simulink model "HighwayLaneFollowingRRTestBench"  (R2023b)
settings: Solver=ode23tb  StartTime=0  StopTime=1000  FixedStep=Ts  RelTol=1e-3
PostLoadFcn:
  | helperSLHighwayLaneFollowingWithRRSetup()
undefined symbols (not defined in the file or in its folder): assessment, camera, Defined, Ego, Lane, m, n, numTargetActors, Ts, User, v_set, vehicleDetectionRange, vehSim3D
libraries: sim3dautolib x6, roadrunnerscenario x4, simulink x4, trackmetricslib x1, sim3dcameralib x1, sim3dprobsensorlib x1, sim3dlib x1, drivingsim3d x1, dspvision x1, drivingscenarioandsensors x1
CloseFcn:
  | helperSLHighwayLaneFollowingWithRRCleanUp()
settings Model: SILPILSystemUnderTest=refmodels  Creator=The MathWorks, Inc.  LastModifiedBy=varun
settings SolverCC: AlgebraicLoopSolver=TrustRegion  MaxZcPerStep=1
settings DataIOCC: SaveOutput=off  DSMLogging=off  SaveTime=off  ReturnWorkspaceOutputs=off
settings OptimizationCC: ReuseModelBlockBuffer=off
settings DebuggingCC: ParameterPrecisionLossMsg=none  UnconnectedInputMsg=warning  UnconnectedOutputMsg=warning  UnconnectedLineMsg=warning  PregeneratedLibrarySubsystemCodeDiagnostic=none  SubsystemReferenceDiagnosticForUnitTest=warning  ArithmeticOperatorsInVariantConditions=warning
settings HardwareCC: ProdLongLongMode=on
settings ModelReferenceCC: EnableRefExpFcnMdlSchedulingChecks=on
settings SFSimCC: SimUseLocalCustomCode=off
settings RTWCC: RTWUseLocalCustomCode=off  DLArmComputeVersion=19.05
settings GRTTargetCC: RTWCAPISignals=on
settings ConfigComp: CovScope=ReferencedModels  CovIncludeTopModel=off

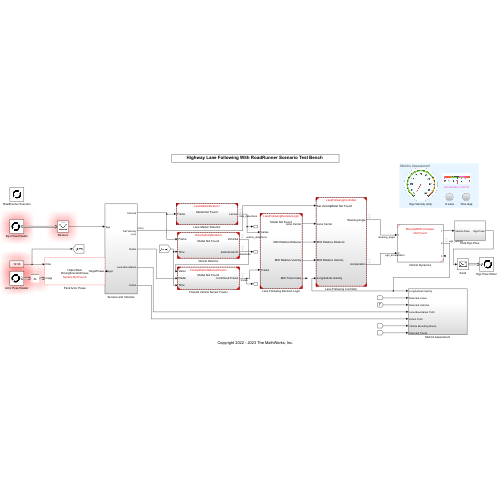
[thumbnail: Simulink's stored preview of the top-level diagram]
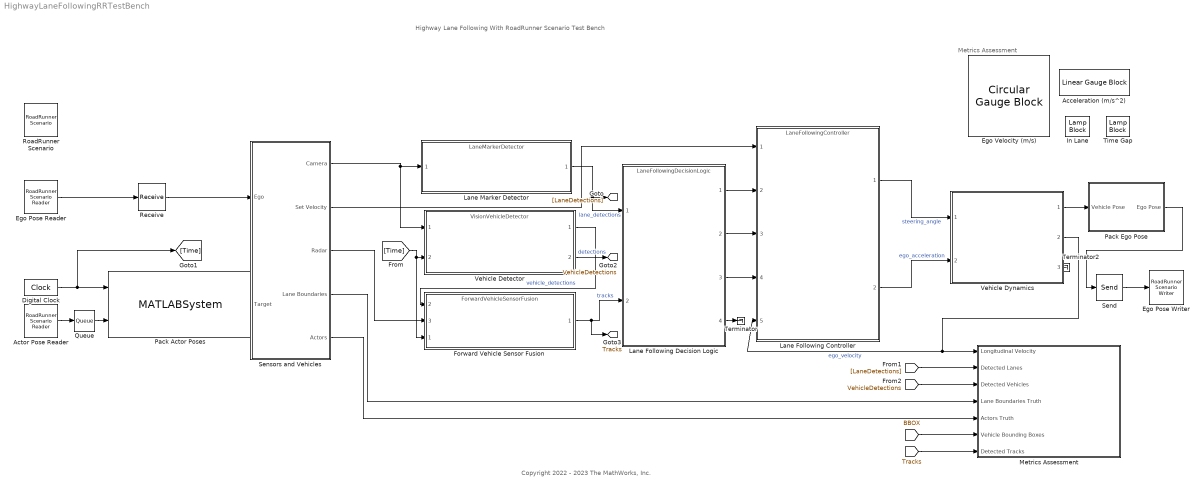
== system HighwayLaneFollowingRRTestBench ==
  note: Highway Lane Following With RoadRunner Scenario Test Bench
  note: Metrics Assessment
  note: Copyright 2022 - 2023 The MathWorks, Inc.
  Acceleration (m/s^2) : LinearGaugeBlock  LabelPosition=Hide  ScaleMin=-6  ScaleMax=6
  Actor Pose Reader : roadrunnerscenario/RoadRunner Scenario Reader  TopicCategory=Actor  ActorCategory=All Types  ActionType=Path Following  EventType=User-Defined  TopicType=Actor Pose (Driving Scenario compatible)  VehicleType=Vehicle Specifications  UserDefinedAction=Action1  UserDefinedEvent=Event1  Filter=None  SensorTopic=Target Poses  LaneBoundaryOutputTopic=Ego-Lane  SensorID=1  SampleTime=Ts
  Digital Clock : DigitalClock  SampleTime=Ts
  Ego Pose Reader : roadrunnerscenario/RoadRunner Scenario Reader  TopicCategory=Actor  ActorCategory=All Types  ActionType=Path Following  EventType=User-Defined  TopicType=Actor Pose (Driving Scenario compatible)  VehicleType=Vehicle Specifications  UserDefinedAction=Action1  UserDefinedEvent=Event1  Filter=Self  SensorTopic=Target Poses  LaneBoundaryOutputTopic=Ego-Lane  SensorID=1  SampleTime=Ts
  Ego Pose Writer : roadrunnerscenario/RoadRunner Scenario Writer  TopicCategory=Actor  ActorCategory=All Types  EventType=Action Complete  UserDefinedEvent=Event1  VehicleType=Vehicle Pose  TopicType=Actor Pose (Driving Scenario compatible)
  Ego Velocity (m/s) : CircularGaugeBlock  LabelPosition=Hide  ScaleMax=50
  Forward Vehicle Sensor Fusion : ModelReference  ModelNameDialog=ForwardVehicleSensorFusion.slx  SimulationMode=Normal  CodeInterface=Top model  ModelReferenceVersion=8.1
      settings: PortSchema="{\"entries\":[{\"content\":{\"sides\":[{\"content\":{\"connectorIds\":[\"In2\",\"In3\",\"In1\"]},\"type\":\"ConnectorPlacement.EquallySpacedRectSide\",\"uuid\":\"7686684e-3ce8-49a8-9c28-78afc562c6cd\"},{\"content\":{\"connectorIds\":[\"Out1\"],\"side\":\"RIGHT\"},\"type\":\"ConnectorPlacement.EquallySpacedRectSide\",\"uuid\":\"c415bca7-2ba8-48d1-9f28-43832dd5ba4e\"},{\"content\":{\"connectorIds\":[],\"side\":\"TOP\"},\"type\":\"ConnectorPlacement.EquallySpacedRectSide\",\"uuid\":\"f22886ed-f0b4-4628-af34-640797a1171b\"}]},\"type\":\"ConnectorPlacement.EquallySpacedConnector\",\"uuid\":\"6b238f4e-3dd4-4f3d-8d3a-ef3e86789fb5\"}],\"packageUris\":[\"http://schema.mathworks.com/mf0/Connector/R2020b\"],\"version\":\"1.0\"}"
  In Lane : LampBlock  LabelPosition=Hide
  Lane Following Controller : ModelReference  ModelNameDialog=LaneFollowingController  SimulationMode=Normal  CodeInterface=Top model  ModelReferenceVersion=8.1
  Lane Following Decision Logic : ModelReference  ModelNameDialog=LaneFollowingDecisionLogic.slx  SimulationMode=Normal  CodeInterface=Top model  ModelReferenceVersion=7.1
  Lane Marker Detector : ModelReference  ModelNameDialog=LaneMarkerDetector.slx  SimulationMode=Normal  CodeInterface=Top model  ModelReferenceVersion=6.1
  Metrics Assessment : Subsystem
  Pack Actor Poses : MATLABSystem  InputPortMessageModes=n,m  System=HelperPackDrivingScenarioPoses  EgoActorID=1  ActorProfiles=actorProfiles  DefaultActorPoses="Simulink.Bus.createMATLABStruct( \"BusActors\" )"
      mask Type: HelperPackDrivingScenarioPoses
      mask Display:
      | disp(['HelperPack' char(10) 'DrivingScenarioPoses']);
      | port_label('input',1,'time');
      | port_label('input',2,'msgs');
      | port_label('output',1,'TargetPoses');
  Pack Ego Pose : Subsystem
  Queue : Queue  InputPortMessageModes=m  OutputPortMessageModes=m  OverwriteOldest=on  Capacity=numTargetActors+2  QueueType=LIFO
  Receive : Receive  InputPortMessageModes=m  UseInternalQueue=off  QueueOverwriting=on  QueueLength=1  QueueType=LIFO  SampleTime=Ts
  RoadRunner Scenario : roadrunnerscenario/RoadRunner Scenario  UserDefinedActions={}  UserDefinedEvents={}
  Send : Send  OutputPortMessageModes=m
  Sensors and Vehicles : Subsystem  VariantControl=1
  Terminator : Terminator
  Terminator2 : Terminator
  Time Gap : LampBlock  LabelPosition=Hide
  Vehicle Detector : ModelReference  ModelNameDialog=VisionVehicleDetector.slx  SimulationMode=Normal  CodeInterface=Top model  ModelReferenceVersion=7.1
  Vehicle Dynamics : Subsystem  VariantControl=Variant2  ReferencedSubsystem=BicycleWithForceInput
  tag scope: Tracks=global, VehicleDetections=global
  wires:
  Ego Pose Reader/1 -> Receive/1
  Lane Following Decision Logic/4 -> Terminator/1
  Digital Clock/1 -> Pack Actor Poses/1, [Time]
  Lane Following Decision Logic/3 -> Lane Following Controller/4
  Vehicle Dynamics/2 -> Lane Following Controller/5, Metrics Assessment/1(Longitudinal Velocity)  "ego_velocity"
  Vehicle Detector/2 -> [VehicleDetections]  "detections"
  Vehicle Detector/1 -> Forward Vehicle Sensor Fusion/2  "vehicle_detections"
  Send/1 -> Ego Pose Writer/1
  Forward Vehicle Sensor Fusion/1 -> [Tracks], Lane Following Decision Logic/2  "tracks"
  Lane Following Decision Logic/2 -> Lane Following Controller/3
  Lane Following Decision Logic/1 -> Lane Following Controller/2
  Lane Following Controller/1 -> Vehicle Dynamics/1  "steering_angle"
  Lane Following Controller/2 -> Vehicle Dynamics/2  "ego_acceleration"
  Sensors and Vehicles/1(Camera) -> Vehicle Detector/1, Lane Marker Detector/1
  Sensors and Vehicles/3(Radar) -> Forward Vehicle Sensor Fusion/3
  Vehicle Dynamics/3 -> Terminator2/1
  Lane Marker Detector/1 -> [LaneDetections], Lane Following Decision Logic/1  "lane_detections"
  Sensors and Vehicles/4(Lane Boundaries) -> Metrics Assessment/4(Lane Boundaries Truth)
  Sensors and Vehicles/2(Set Velocity) -> Lane Following Controller/1
  Vehicle Dynamics/1 -> Pack Ego Pose/1(Vehicle Pose)
  Receive/1 -> Sensors and Vehicles/1(Ego)
  Actor Pose Reader/1 -> Queue/1
  Pack Ego Pose/1(Ego Pose) -> Send/1
  Queue/1 -> Pack Actor Poses/2
  [Time] -> Forward Vehicle Sensor Fusion/1, Vehicle Detector/2
  Pack Actor Poses/1 -> Sensors and Vehicles/2(Target)
  [LaneDetections] -> Metrics Assessment/2(Detected Lanes)
  [VehicleDetections] -> Metrics Assessment/3(Detected Vehicles)
  [Tracks] -> Metrics Assessment/7(Detected Tracks)
  Sensors and Vehicles/5(Actors) -> Metrics Assessment/5(Actors Truth)
  [BBOX] -> Metrics Assessment/6(Vehicle Bounding Boxes)

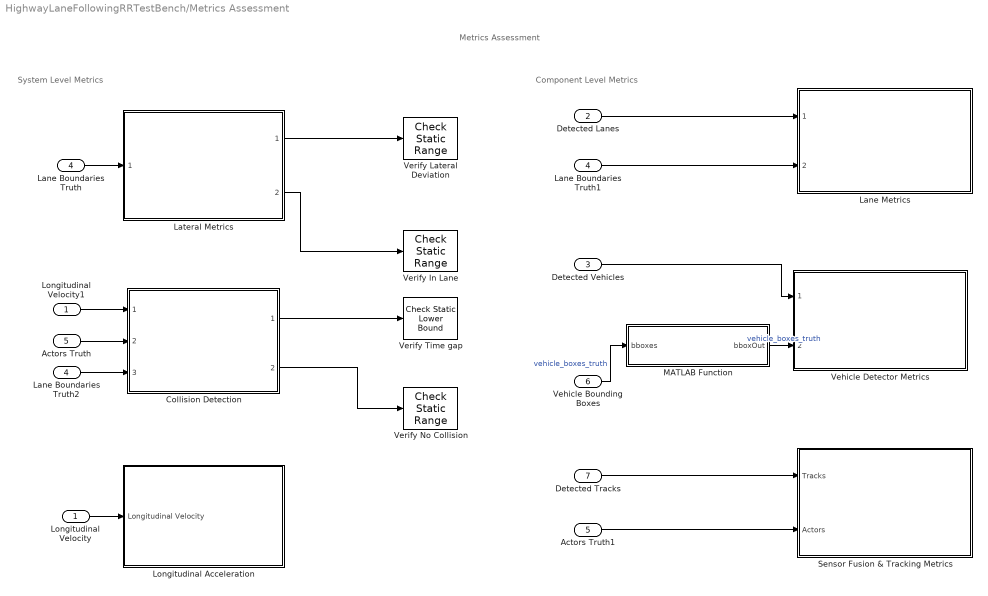
== system HighwayLaneFollowingRRTestBench/Metrics Assessment ==
  note: System Level Metrics
  note: Component Level Metrics
  note: Metrics Assessment
  Longitudinal Velocity : Inport
  Detected Lanes : Inport  Port=2
  Detected Vehicles : Inport  Port=3
  Lane Boundaries Truth : Inport  Port=4
  Actors Truth : Inport  Port=5
  Vehicle Bounding Boxes : Inport  Port=6
  Detected Tracks : Inport  Port=7
  " Vehicle Detector Metrics" : Subsystem  ReferencedSubsystem=VehicleDetectorMetrics
  Actors Truth1 : InportShadow  Port=5
  Collision Detection : Subsystem  ReferencedSubsystem=CollisionDetection
  Lane Boundaries Truth1 : InportShadow  Port=4
  Lane Boundaries Truth2 : InportShadow  Port=4
  Lane Metrics : Subsystem  ReferencedSubsystem=LaneMetrics
  Lateral Metrics : Subsystem  ReferencedSubsystem=LateralMetrics
  Longitudinal Acceleration : Subsystem
  Longitudinal Velocity1 : InportShadow
  MATLAB Function : MATLAB Function  TreatAsAtomicUnit=on  mask{camera=camera, range=vehicleDetectionRange}
  Sensor Fusion & Tracking Metrics : Subsystem
  Verify In Lane : simulink/Model Verification/Check  Static Range  Description=1 <= u <= 1  max=1  max_included=on  min=1  min_included=on  enabled=on  stopWhenAssertionFail=on  export=off  icon=graphic
  Verify Lateral Deviation : simulink/Model Verification/Check  Static Range  Description=-assessment.LateralDeviationMax <= u <= assessment.LateralDeviationMax  max=assessment.LateralDeviationMax  max_included=on  min=-assessment.LateralDeviationMax  min_included=on  enabled=on  stopWhenAssertionFail=on  export=off  icon=graphic
      settings: AttributesFormatString=|
      | ---------------------------------------
      | max = %<max>
      | min = %<min>
  Verify No Collision : simulink/Model Verification/Check  Static Range  Description=0 <= u <= 0  max=0  max_included=on  min=0  min_included=on  enabled=on  stopWhenAssertionFail=on  export=off  icon=graphic
  Verify Time gap : simulink/Model Verification/Check Static  Lower Bound  Description=assessment.TimeGap <= u  min=assessment.TimeGap  min_included=on  enabled=on  stopWhenAssertionFail=on  export=off  icon=graphic
      settings: AttributesFormatString=|
      | ---------------------------------------
      | min = %<min>
  wires:
  Lane Boundaries Truth/1 -> Lateral Metrics/1
  Collision Detection/1 -> Verify Time gap/1
  Lateral Metrics/1 -> Verify Lateral Deviation/1
  Collision Detection/2 -> Verify No Collision/1
  Longitudinal Velocity/1 -> Longitudinal Acceleration/1(Longitudinal Velocity)
  Actors Truth/1 -> Collision Detection/2
  Lateral Metrics/2 -> Verify In Lane/1
  Lane Boundaries Truth2/1 -> Collision Detection/3
  Detected Lanes/1 -> Lane Metrics/1
  Detected Vehicles/1 -> " Vehicle Detector Metrics"/1
  Vehicle Bounding Boxes/1 -> MATLAB Function/1(bboxes)  "vehicle_boxes_truth"
  Lane Boundaries Truth1/1 -> Lane Metrics/2
  Longitudinal Velocity1/1 -> Collision Detection/1
  MATLAB Function/1(bboxOut) -> " Vehicle Detector Metrics"/2  "vehicle_boxes_truth"
  Detected Tracks/1 -> Sensor Fusion & Tracking Metrics/1(Tracks)
  Actors Truth1/1 -> Sensor Fusion & Tracking Metrics/2(Actors)

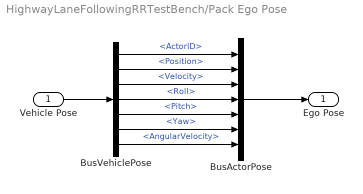
== system HighwayLaneFollowingRRTestBench/Pack Ego Pose ==
  Vehicle Pose : Inport
  BusActorPose : BusCreator  Inputs=7  OutDataTypeStr=Bus: BusActorPose  NonVirtualBus=on
      settings: InheritFromInputs=off
  BusVehiclePose : BusSelector  OutputSignals=ActorID,Position,Velocity,Roll,Pitch,Yaw,AngularVelocity
  Ego Pose : Outport
  wires:
  BusVehiclePose/4 -> BusActorPose/4  "<Roll>"
  BusVehiclePose/3 -> BusActorPose/3  "<Velocity>"
  BusVehiclePose/1 -> BusActorPose/1  "<ActorID>"
  BusVehiclePose/2 -> BusActorPose/2  "<Position>"
  BusVehiclePose/7 -> BusActorPose/7  "<AngularVelocity>"
  BusVehiclePose/6 -> BusActorPose/6  "<Yaw>"
  BusVehiclePose/5 -> BusActorPose/5  "<Pitch>"
  Vehicle Pose/1 -> BusVehiclePose/1
  BusActorPose/1 -> Ego Pose/1

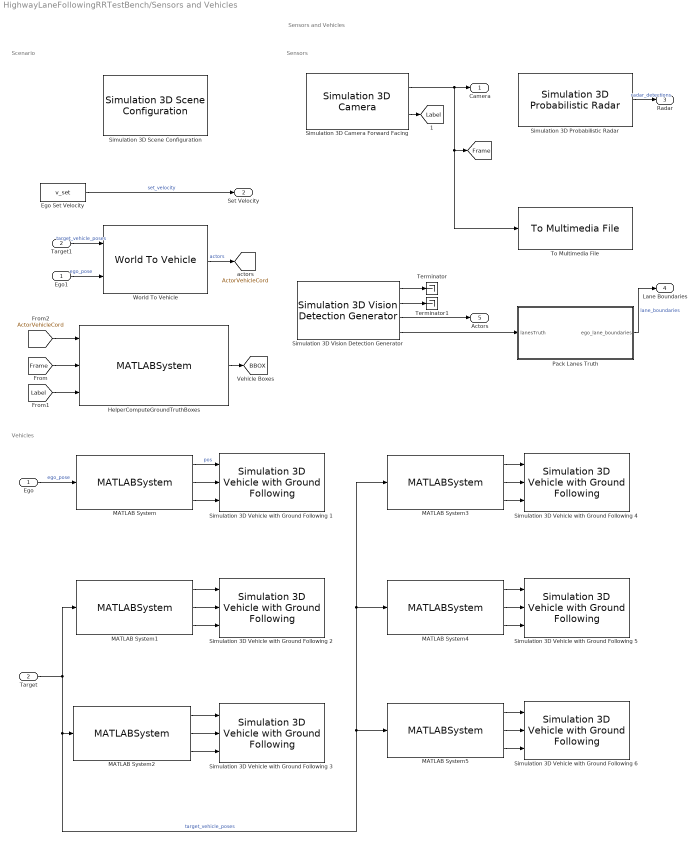
== system HighwayLaneFollowingRRTestBench/Sensors and Vehicles ==
  note: Scenario
  note: Vehicles
  note: Sensors and Vehicles
  note: Sensors
  Ego : Inport
  Target : Inport  Port=2
  Ego Set Velocity : Constant  Value=v_set  SampleTime=Ts
  Ego1 : InportShadow
  HelperComputeGroundTruthBoxes : MATLABSystem  System=HelperComputeGroundTruthBoxes  VehicleDimensions=actorDimensions  Camera=camera  SimulateUsing=Interpreted execution
      mask Type: HelperComputeGroundTruthBoxes
      mask Display:
      | disp('HelperComputeGroundTruthBoxes');
      | port_label('input',1,'actorPositions');
      | port_label('input',2,'frame');
      | port_label('input',3,'labelledFrame');
      | port_label('output',1,'BBoxes');
  MATLAB System : MATLABSystem  System=HelperConvertDSPoseToSim3D  ActorProfiles=actorProfiles  ActorIDToConvert=1  SimulateUsing=Interpreted execution
      mask Type: HelperConvertDSPoseToSim3D
      mask Display:
      | disp(['HelperConvert' char(10) 'DSPoseToSim3D' char(10) 'ActorID: 1']);
      | port_label('input',1,'Actor');
      | port_label('output',1,'X');
      | port_label('output',2,'Y');
      | port_label('output',3,'Yaw');
  MATLAB System1 : MATLABSystem  System=HelperConvertDSPoseToSim3D  ActorProfiles=actorProfiles  ActorIDToConvert=2  SimulateUsing=Interpreted execution
      mask Type: HelperConvertDSPoseToSim3D
      mask Display:
      | disp(['HelperConvert' char(10) 'DSPoseToSim3D' char(10) 'ActorID: 2']);
      | port_label('input',1,'Actor');
      | port_label('output',1,'X');
      | port_label('output',2,'Y');
      | port_label('output',3,'Yaw');
  MATLAB System2 : MATLABSystem  System=HelperConvertDSPoseToSim3D  ActorProfiles=actorProfiles  ActorIDToConvert=3  SimulateUsing=Interpreted execution
      mask Type: HelperConvertDSPoseToSim3D
      mask Display:
      | disp(['HelperConvert' char(10) 'DSPoseToSim3D' char(10) 'ActorID: 3']);
      | port_label('input',1,'Actor');
      | port_label('output',1,'X');
      | port_label('output',2,'Y');
      | port_label('output',3,'Yaw');
  MATLAB System3 : MATLABSystem  System=HelperConvertDSPoseToSim3D  ActorProfiles=actorProfiles  ActorIDToConvert=4  SimulateUsing=Interpreted execution
      mask Type: HelperConvertDSPoseToSim3D
      mask Display:
      | disp(['HelperConvert' char(10) 'DSPoseToSim3D' char(10) 'ActorID: 4']);
      | port_label('input',1,'Actor');
      | port_label('output',1,'X');
      | port_label('output',2,'Y');
      | port_label('output',3,'Yaw');
  MATLAB System4 : MATLABSystem  System=HelperConvertDSPoseToSim3D  ActorProfiles=actorProfiles  ActorIDToConvert=5  SimulateUsing=Interpreted execution
      mask Type: HelperConvertDSPoseToSim3D
      mask Display:
      | disp(['HelperConvert' char(10) 'DSPoseToSim3D' char(10) 'ActorID: 5']);
      | port_label('input',1,'Actor');
      | port_label('output',1,'X');
      | port_label('output',2,'Y');
      | port_label('output',3,'Yaw');
  MATLAB System5 : MATLABSystem  System=HelperConvertDSPoseToSim3D  ActorProfiles=actorProfiles  ActorIDToConvert=6  SimulateUsing=Interpreted execution
      mask Type: HelperConvertDSPoseToSim3D
      mask Display:
      | disp(['HelperConvert' char(10) 'DSPoseToSim3D' char(10) 'ActorID: 6']);
      | port_label('input',1,'Actor');
      | port_label('output',1,'X');
      | port_label('output',2,'Y');
      | port_label('output',3,'Yaw');
  Pack Lanes Truth : MATLAB Function  TreatAsAtomicUnit=on  mask{detStructObj=Simulink.Bus.createMATLABStruct('LaneSensor'), boundariesStructObj=Simulink.Bus.createMATLABStruct('BusLaneBoundaries')}
      mask prompts: detStructObj "Output lane detections struct"; boundariesStructObj "Output lane boundaries struct"
  Simulation 3D Camera Forward Facing : sim3dcameralib/Simulation 3D Camera  Priority=1  sensorTag=Sim3dSensor1  sensorId=1  sensorName=Sim3dSensor1  vehTagList={'Scene Origin';'SimulinkVehicle1';'SimulinkVehicle2';'SimulinkVehicle3';'SimulinkVehicle4';'SimulinkVehicle5';'SimulinkVehicle6'}  vehTag=Scene Origin  mountLoc=Origin  offsetFlag=on  tmountOffset=[0,-1,1]  extTmount=off  rmountOffset=[0,0,-90]  extRmount=off  FocalLength=camera.FocalLength  OpticalCenter=camera.PrincipalPoint  ImageSize=camera.ImageSize  RadialDistortion=[0, 0]  TangentialDistortion=[0, 0]  SensorSkew=0  DepthOutportEnabled=off  SemanticOutportEnabled=on  TransformOutportEnabled=off  SampleTime=-1  mountPoint=[0 1 1]  mountOrientation=[0 0 90]  aMode=3  ID=1
      settings: LibrarySourceBlock=drivingsim3d/Simulation 3D Camera
      settings: AttributesFormatString=|
      | -------------------------------------
      | ImageSize = %<ImageSize>
      | OpticalCenter = %<OpticalCenter>
      | FocalLength = %<FocalLength>
      | RadialDistortion = %<RadialDistortion>
      | mountLoc = %<mountLoc>
      | tmountOffset = %<tmountOffset>
      | rmountOffset = %<rmountOffset>
      | Priority = %<Priority>
  Simulation 3D Probabilistic Radar : sim3dprobsensorlib/Simulation 3D Probabilistic Radar  Priority=1  sensorTag=Sim3dSensor2  sensorId=2  sensorName=Sim3dSensor2  vehTagList={'Scene Origin';'SimulinkVehicle1';'SimulinkVehicle2';'SimulinkVehicle3';'SimulinkVehicle4';'SimulinkVehicle5';'SimulinkVehicle6'}  vehTag=SimulinkVehicle1  mountLoc=Origin  offsetFlag=on  tmountOffset=radar.PositionSim3d  rmountOffset=radar.Rotation  AzimuthResolution=0.8  ElevationResolution=8  RangeResolution=1  RangeRateResolution=1  AzimuthBiasFraction=0.1  ElevationBiasFraction=0.1  RangeBiasFraction=0.05  RangeRateBiasFraction=0.05  FieldOfView=radar.FieldOfView  DetectionRange=radar.DetectionRanges  RangeRateLimits=[ -100, 100 ]  DetectionProbability=0.9  FalseAlarmRate=1e-6  ReferenceRange=150  ReferenceRCS=0  HasElevation=off  HasRangeRate=on  HasNoise=off  HasFalseAlarms=off  InitialSeedSource=Repeatable  InitialSeed=0  MaxNumDetections=50  DetectionCoordinates=Sensor spherical  SpecifyOutputBusName=off  BusName=BusSimulation3DRadarTruthSensor  SampleTime=-1  mountPoint=[0 0 1]  mountOrientation=[0 0 0]  aMode=3  ID=2
      settings: LibrarySourceBlock=drivingsim3d/Simulation 3D Probabilistic Radar
      settings: AttributesFormatString=|
      | -------------------------------------
      | FieldOfView = %<FieldOfView>
      | AzimuthResolution = %<AzimuthResolution>
      | DetectionCoordinates = %<DetectionCoordinates>
      | mountLoc = %<mountLoc>
      | tmountOffset = %<tmountOffset>
      | rmountOffset = %<rmountOffset>
      | Priority = %<Priority>
  Simulation 3D Scene Configuration : sim3dlib/Simulation 3D Scene Configuration  Priority=0  ProjectFormat=RoadRunner  SceneDesc=Large parking lot  ProjectName=C:\Program Files\MATLAB\R2023b\toolbox\shared\sim3d_projects\automotive_project_windows\UE\WindowsNoEditor\VehicleSimulation.exe  ScenePath=/Game/Maps/HwStrght  RoadRunnerProjectPath=C:\Users\varun\ME599\AutoPark\AutoPark\Exports\AutoPark.xosc  EnableOpenDRIVE=off  vehTagList={'Custom';'Scene Origin';'SimulinkVehicle1';'SimulinkVehicle2';'SimulinkVehicle3';'SimulinkVehicle4';'SimulinkVehicle5';'SimulinkVehicle6'}  vehTag=Scene Origin  FreeCameraInitialTranslation=[0, 0, 0]  FreeCameraDefaultInitialTranslation=[-6, 0, 2]  FreeCameraInitialRotation=[0, 0, 0]  FreeCameraDefaultInitialRotation=[0, -15, 0]  OpVisEn=off  Ts=Ts  EnableWindow=on  EnableRemoteAccess=off  EnableWeather=off  SunAltitude=40.0  SunAzimuth=90  clouds=10  wind=1  fog=0  rain=0  EnableGeospatial=off  OriginHeight=200  OriginLatitude=40.744652  OriginLongitude=-73.988864  MapStyle=Aerial  AdditionalAssetIDs=[]  UseAdvancedSunSky=off  SolarTime=11  TimeZone=-5  Day=21  Month=9  Year=2022  UseDaylightSavingTime=on  DSTStartDay=10  DSTStartMonth=3  DSTEndDay=3  DSTEndMonth=11  DSTSwitchHour=2  sensorTag=MainCamera3  sensorId=3  sensorName=MainCamera3  mountLoc=Origin  offsetFlag=off  tmountOffset=[0, 0, 0]  rmountOffset=[0, 0, 0]  HorizontalResolution=1280  VerticalResolution=720  HorizontalFOV=60  mountPoint=[0 0 0]  mountOrientation=[0 0 0]  aMode=3  ID=3  GeoTrigger=Inactive
      settings: LibrarySourceBlock=drivingsim3d/Simulation 3D Scene Configuration
      settings: AttributesFormatString=|
      | -------------------------------------
      | SceneName = %<SceneDesc>
      | Priority = %<Priority>
  Simulation 3D Vehicle with Ground Following 1 : sim3dautolib/Simulation 3D Vehicle with Ground Following  Priority=-1  PassVehMesh=Sedan  MeshPath=/MathWorksSimulation/Vehicles/Muscle/Meshes/SK_MuscleCar.SK_MuscleCar  TrackWidth=1.9  WheelBase=3  WheelRadius=0.35  VehColor=Blue  InitialPos=vehSim3D(1).InitialPos  InitialRot=vehSim3D(1).InitialRot  ActorName=SimulinkVehicle1  SampleTime=-1  ActorType=SimulinkVehicle  ID=1  aMode=3  ActorTag=SimulinkVehicle1  CoordinateScheme=ISO  VehLightsControl=off  HeadlightColor=[ 1, 1, 1 ]  HighBeamIntensity=100000  LowBeamIntensity=60000  HighBeamConeAngle=70  LowBeamConeAngle=70  LeftHeadlightOrientation=[ 0, 0 ]  RightHeadlightOrientation=[ 0, 0 ]  BrakelightIntensity=500  ReverselightIntensity=500  SignallightIntensity=500  SignallightPeriod=1  SignalPulseWidth=50  TransformOutportEnabled=off
      settings: LibrarySourceBlock=drivingsim3d/Simulation 3D Vehicle with Ground Following
      settings: AttributesFormatString=|
      | --------------------------------------
      | ActorName = %<ActorName>
      | PassVehMesh = %<PassVehMesh>
      | VehColor = %<VehColor>
      | InitialPos = %<InitialPos>
      | InitialRot = %<InitialRot>
      | Priority = %<Priority>
  Simulation 3D Vehicle with Ground Following 2 : sim3dautolib/Simulation 3D Vehicle with Ground Following  Priority=-1  PassVehMesh=Sedan  MeshPath=/MathWorksSimulation/Vehicles/Muscle/Meshes/SK_MuscleCar.SK_MuscleCar  TrackWidth=1.9  WheelBase=3  WheelRadius=0.35  VehColor=Red  InitialPos=vehSim3D(2).InitialPos  InitialRot=vehSim3D(2).InitialRot  ActorName=SimulinkVehicle2  SampleTime=-1  ActorType=SimulinkVehicle  ID=2  aMode=3  ActorTag=SimulinkVehicle2  CoordinateScheme=ISO  VehLightsControl=off  HeadlightColor=[ 1, 1, 1 ]  HighBeamIntensity=100000  LowBeamIntensity=60000  HighBeamConeAngle=70  LowBeamConeAngle=70  LeftHeadlightOrientation=[ 0, 0 ]  RightHeadlightOrientation=[ 0, 0 ]  BrakelightIntensity=500  ReverselightIntensity=500  SignallightIntensity=500  SignallightPeriod=1  SignalPulseWidth=50  TransformOutportEnabled=off
      settings: LibrarySourceBlock=drivingsim3d/Simulation 3D Vehicle with Ground Following
      settings: AttributesFormatString=|
      | --------------------------------------
      | ActorName = %<ActorName>
      | PassVehMesh = %<PassVehMesh>
      | VehColor = %<VehColor>
      | InitialPos = %<InitialPos>
      | InitialRot = %<InitialRot>
      | Priority = %<Priority>
  Simulation 3D Vehicle with Ground Following 3 : sim3dautolib/Simulation 3D Vehicle with Ground Following  Priority=-1  PassVehMesh=Sedan  MeshPath=/MathWorksSimulation/Vehicles/Muscle/Meshes/SK_MuscleCar.SK_MuscleCar  TrackWidth=1.9  WheelBase=3  WheelRadius=0.35  VehColor=Black  InitialPos=vehSim3D(3).InitialPos  InitialRot=vehSim3D(3).InitialRot  ActorName=SimulinkVehicle3  SampleTime=-1  ActorType=SimulinkVehicle  ID=3  aMode=3  ActorTag=SimulinkVehicle3  CoordinateScheme=ISO  VehLightsControl=off  HeadlightColor=[ 1, 1, 1 ]  HighBeamIntensity=100000  LowBeamIntensity=60000  HighBeamConeAngle=70  LowBeamConeAngle=70  LeftHeadlightOrientation=[ 0, 0 ]  RightHeadlightOrientation=[ 0, 0 ]  BrakelightIntensity=500  ReverselightIntensity=500  SignallightIntensity=500  SignallightPeriod=1  SignalPulseWidth=50  TransformOutportEnabled=off
      settings: LibrarySourceBlock=drivingsim3d/Simulation 3D Vehicle with Ground Following
      settings: AttributesFormatString=|
      | --------------------------------------
      | ActorName = %<ActorName>
      | PassVehMesh = %<PassVehMesh>
      | VehColor = %<VehColor>
      | InitialPos = %<InitialPos>
      | InitialRot = %<InitialRot>
      | Priority = %<Priority>
  Simulation 3D Vehicle with Ground Following 4 : sim3dautolib/Simulation 3D Vehicle with Ground Following  Priority=-1  PassVehMesh=Sedan  MeshPath=/MathWorksSimulation/Vehicles/Muscle/Meshes/SK_MuscleCar.SK_MuscleCar  TrackWidth=1.9  WheelBase=3  WheelRadius=0.35  VehColor=Orange  InitialPos=vehSim3D(4).InitialPos  InitialRot=vehSim3D(4).InitialRot  ActorName=SimulinkVehicle4  SampleTime=-1  ActorType=SimulinkVehicle  ID=4  aMode=3  ActorTag=SimulinkVehicle4  CoordinateScheme=ISO  VehLightsControl=off  HeadlightColor=[ 1, 1, 1 ]  HighBeamIntensity=100000  LowBeamIntensity=60000  HighBeamConeAngle=70  LowBeamConeAngle=70  LeftHeadlightOrientation=[ 0, 0 ]  RightHeadlightOrientation=[ 0, 0 ]  BrakelightIntensity=500  ReverselightIntensity=500  SignallightIntensity=500  SignallightPeriod=1  SignalPulseWidth=50  TransformOutportEnabled=off
      settings: LibrarySourceBlock=drivingsim3d/Simulation 3D Vehicle with Ground Following
      settings: AttributesFormatString=|
      | --------------------------------------
      | ActorName = %<ActorName>
      | PassVehMesh = %<PassVehMesh>
      | VehColor = %<VehColor>
      | InitialPos = %<InitialPos>
      | InitialRot = %<InitialRot>
      | Priority = %<Priority>
  Simulation 3D Vehicle with Ground Following 5 : sim3dautolib/Simulation 3D Vehicle with Ground Following  Priority=-1  PassVehMesh=Sedan  MeshPath=/MathWorksSimulation/Vehicles/Muscle/Meshes/SK_MuscleCar.SK_MuscleCar  TrackWidth=1.9  WheelBase=3  WheelRadius=0.35  VehColor=Green  InitialPos=vehSim3D(5).InitialPos  InitialRot=vehSim3D(5).InitialRot  ActorName=SimulinkVehicle5  SampleTime=-1  ActorType=SimulinkVehicle  ID=5  aMode=3  ActorTag=SimulinkVehicle5  CoordinateScheme=ISO  VehLightsControl=off  HeadlightColor=[ 1, 1, 1 ]  HighBeamIntensity=100000  LowBeamIntensity=60000  HighBeamConeAngle=70  LowBeamConeAngle=70  LeftHeadlightOrientation=[ 0, 0 ]  RightHeadlightOrientation=[ 0, 0 ]  BrakelightIntensity=500  ReverselightIntensity=500  SignallightIntensity=500  SignallightPeriod=1  SignalPulseWidth=50  TransformOutportEnabled=off
      settings: LibrarySourceBlock=drivingsim3d/Simulation 3D Vehicle with Ground Following
      settings: AttributesFormatString=|
      | --------------------------------------
      | ActorName = %<ActorName>
      | PassVehMesh = %<PassVehMesh>
      | VehColor = %<VehColor>
      | InitialPos = %<InitialPos>
      | InitialRot = %<InitialRot>
      | Priority = %<Priority>
  Simulation 3D Vehicle with Ground Following 6 : sim3dautolib/Simulation 3D Vehicle with Ground Following  Priority=-1  PassVehMesh=Sedan  MeshPath=/MathWorksSimulation/Vehicles/Muscle/Meshes/SK_MuscleCar.SK_MuscleCar  TrackWidth=1.9  WheelBase=3  WheelRadius=0.35  VehColor=Blue  InitialPos=vehSim3D(6).InitialPos  InitialRot=vehSim3D(6).InitialRot  ActorName=SimulinkVehicle6  SampleTime=-1  ActorType=SimulinkVehicle  ID=6  aMode=3  ActorTag=SimulinkVehicle6  CoordinateScheme=ISO  VehLightsControl=off  HeadlightColor=[ 1, 1, 1 ]  HighBeamIntensity=100000  LowBeamIntensity=60000  HighBeamConeAngle=70  LowBeamConeAngle=70  LeftHeadlightOrientation=[ 0, 0 ]  RightHeadlightOrientation=[ 0, 0 ]  BrakelightIntensity=500  ReverselightIntensity=500  SignallightIntensity=500  SignallightPeriod=1  SignalPulseWidth=50  TransformOutportEnabled=off
      settings: LibrarySourceBlock=drivingsim3d/Simulation 3D Vehicle with Ground Following
      settings: AttributesFormatString=|
      | --------------------------------------
      | ActorName = %<ActorName>
      | PassVehMesh = %<PassVehMesh>
      | VehColor = %<VehColor>
      | InitialPos = %<InitialPos>
      | InitialRot = %<InitialRot>
      | Priority = %<Priority>
  Simulation 3D Vision Detection Generator : drivingsim3d/Simulation 3D Vision Detection Generator  Priority=1  VariantControl=Choice  sensorTag=Sim3dSensor255  sensorId=3  sensorName=Sim3dSensor3  vehTagList={'Scene Origin';'SimulinkVehicle1';'SimulinkVehicle2';'SimulinkVehicle3';'SimulinkVehicle4';'SimulinkVehicle5';'SimulinkVehicle6'}  vehTag=SimulinkVehicle1  mountLoc=Origin  offsetFlag=on  tmountOffset=[0,-1,1]  rmountOffset=[0,0,0]  DetectorOutput=Lanes and objects  MaxNumDetections=5  MaxNumLanes=30  laneSampleDistances=0:0.5:70  BusNameSource=Property  BusName=BusObjectDetections  BusName2Source=Property  BusName2=BusLaneDetections  MaxRange=camera.DetectionRanges(2)  BoundingBoxAccuracy=5  ProcessNoiseIntensity=5  MaxSpeed=50  MaxAllowedOcclusion=0.5  MinObjectImageSize=camera.MinObjectImageSize  DetectionProbability=1  FalsePositivesPerImage=0  MinLaneImageSize=[ 20, 3 ]  LaneBoundaryAccuracy=3  HasNoise=off  InitialSeedSource=Repeatable  InitialSeed=1  uniqueActorIdentifier=[]  actorClassInteger=0  cuboidLength=4.7  cuboidWidth=1.8  cuboidHeight=1.4  rotationalCenter={[-1.35, 0, 0]}  focalLength=camera.FocalLength  opticalCenter=camera.PrincipalPoint  imageSize=camera.ImageSize  radialDistortionCoefficients=[0, 0]  tangentialDistortionCoefficients=[0, 0]  cameraAxisSkew=0  actorTruthOutportEnabled=on  laneTruthOutportEnabled=on  SampleTime=-1  checkedSampleTime=0.1  mountPoint=[0 1 1]  mountOrientation=[0 0 0]  aMode=3  ID=3
      settings: AttributesFormatString=|
      | imageSize = %<imageSize>
      | opticalCenter = %<opticalCenter>
      | focalLength = %<focalLength>
      | radialDistortionCoefficients = %<radialDistortionCoefficients>
      | mountLoc = %<mountLoc>
      | tmountOffset = %<tmountOffset>
      | rmountOffset = %<rmountOffset>
  Target1 : InportShadow  Port=2
  Terminator : Terminator
  Terminator1 : Terminator
  To Multimedia File : dspvision/To Multimedia File  outputFilename=forwardFacingCamera.mp4  streamSelection=Video only  videoCompressor=None (uncompressed)  audioCompressor=None (uncompressed)  imagePorts=One multidimensional signal  fileType=MPEG4  audioDatatype=Determine from input data type  fourcc=RGB  videoQuality=75  mj2000CompFactor=10
  World To Vehicle : drivingscenarioandsensors/World To Vehicle  BusNameSource=Auto  BusName=BusActors  SimulateUsing=Interpreted execution
  Camera : Outport  VectorParamsAs1DForOutWhenUnconnected=off
  Set Velocity : Outport  Port=2  Unit=m/s  VectorParamsAs1DForOutWhenUnconnected=off
  Radar : Outport  Port=3  VectorParamsAs1DForOutWhenUnconnected=off
  Lane Boundaries : Outport  Port=4
  Actors : Outport  Port=5
  tag scope: ActorVehicleCord=global, BBOX=global, Frame=global, Label=global
  wires:
  MATLAB System/2 -> Simulation 3D Vehicle with Ground Following 1/2
  MATLAB System/1 -> Simulation 3D Vehicle with Ground Following 1/1  "pos"
  MATLAB System/3 -> Simulation 3D Vehicle with Ground Following 1/3
  MATLAB System1/2 -> Simulation 3D Vehicle with Ground Following 2/2
  MATLAB System1/1 -> Simulation 3D Vehicle with Ground Following 2/1
  MATLAB System1/3 -> Simulation 3D Vehicle with Ground Following 2/3
  Simulation 3D Probabilistic Radar/1 -> Radar/1  "radar_detections"
  Simulation 3D Camera Forward Facing/1 -> To Multimedia File/1, [Frame], Camera/1
  MATLAB System3/2 -> Simulation 3D Vehicle with Ground Following 4/2
  MATLAB System3/3 -> Simulation 3D Vehicle with Ground Following 4/3
  MATLAB System2/2 -> Simulation 3D Vehicle with Ground Following 3/2
  MATLAB System3/1 -> Simulation 3D Vehicle with Ground Following 4/1
  MATLAB System2/3 -> Simulation 3D Vehicle with Ground Following 3/3
  MATLAB System2/1 -> Simulation 3D Vehicle with Ground Following 3/1
  MATLAB System4/3 -> Simulation 3D Vehicle with Ground Following 5/3
  MATLAB System5/2 -> Simulation 3D Vehicle with Ground Following 6/2
  MATLAB System5/3 -> Simulation 3D Vehicle with Ground Following 6/3
  MATLAB System5/1 -> Simulation 3D Vehicle with Ground Following 6/1
  MATLAB System4/2 -> Simulation 3D Vehicle with Ground Following 5/2
  MATLAB System4/1 -> Simulation 3D Vehicle with Ground Following 5/1
  Ego Set Velocity/1 -> Set Velocity/1  "set_velocity"
  Target/1 -> MATLAB System1/1, MATLAB System5/1, MATLAB System4/1, MATLAB System3/1, MATLAB System2/1  "target_vehicle_poses"
  Simulation 3D Vision Detection Generator/1 -> Terminator/1
  Pack Lanes Truth/1(ego_lane_boundaries) -> Lane Boundaries/1  "lane_boundaries"
  Ego1/1 -> World To Vehicle/2  "ego_pose"
  Target1/1 -> World To Vehicle/1  "target_vehicle_poses"
  World To Vehicle/1 -> [ActorVehicleCord]  "actors"
  Ego/1 -> MATLAB System/1  "ego_pose"
  HelperComputeGroundTruthBoxes/1 -> [BBOX]
  [Label] -> HelperComputeGroundTruthBoxes/3
  [Frame] -> HelperComputeGroundTruthBoxes/2
  [ActorVehicleCord] -> HelperComputeGroundTruthBoxes/1
  Simulation 3D Camera Forward Facing/2 -> [Label]
  Simulation 3D Vision Detection Generator/3 -> Actors/1
  Simulation 3D Vision Detection Generator/2 -> Terminator1/1
  Simulation 3D Vision Detection Generator/4 -> Pack Lanes Truth/1(lanesTruth)

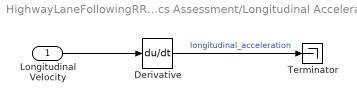
== system HighwayLaneFollowingRRTestBench/Metrics Assessment/Longitudinal Acceleration ==
  Longitudinal Velocity : Inport
  Derivative : Derivative
  Terminator : Terminator
  wires:
  Derivative/1 -> Terminator/1  "longitudinal_acceleration"
  Longitudinal Velocity/1 -> Derivative/1

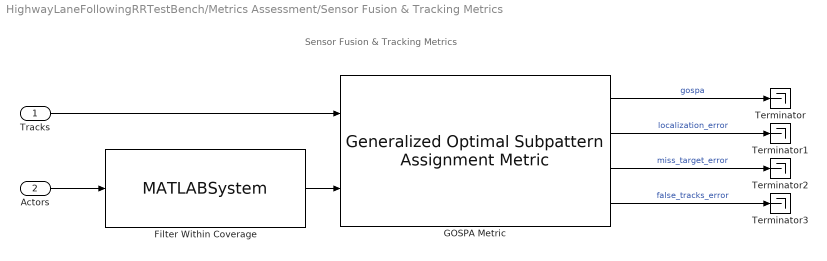
== system HighwayLaneFollowingRRTestBench/Metrics Assessment/Sensor Fusion & Tracking Metrics ==
  note: Sensor Fusion & Tracking Metrics
  Tracks : Inport
  Actors : Inport  Port=2
  Filter Within Coverage : MATLABSystem  System=HelperFilterWithinCoverage  Camera=camera  Radar=radar  OutputBusName=BusSimulation3DActors1
      mask Type: HelperFilterWithinCoverage
      mask Display:
      | disp('HelperFilterWithinCoverage');
      | port_label('input',1,'actors');
      | port_label('output',1,'truth');
  GOSPA Metric : trackmetricslib/Generalized Optimal Subpattern Assignment Metric  CutoffDistance=cutOffDistance  Order=order  Alpha=alpha  Distance=custom  MotionModel=constvel  DistanceFcn=helperComputeDistanceToTruth  SwitchingPenalty=switchingPenalty  SimulateUsing=Interpreted execution  HasAssignmentInput=off  EnableGOSPAOutput=off  EnableSwitchingGOSPAOutput=off  EnableLocalizationGOSPAOutput=on  EnableMissedTargetGOSPAOutput=on  EnableFalseTrackGOSPAOutput=on  TrackFormat=objectTrack  TruthFormat=Actor
  Terminator{,1..3} (4 alike) : Terminator
  wires:
  GOSPA Metric/1 -> Terminator/1  "gospa"
  GOSPA Metric/2 -> Terminator1/1  "localization_error"
  GOSPA Metric/3 -> Terminator2/1  "miss_target_error"
  Tracks/1 -> GOSPA Metric/1
  Actors/1 -> Filter Within Coverage/1
  GOSPA Metric/4 -> Terminator3/1  "false_tracks_error"
  Filter Within Coverage/1 -> GOSPA Metric/2

== matlab function HighwayLaneFollowingRRTestBench/Sensors and Vehicles/Pack Lanes Truth ==
  data: lanesTruth input; ego_lane_boundaries output Bus: BusLaneBoundaries; boundariesStructObj parameter
function ego_lane_boundaries = packLanesTruth(lanesTruth, boundariesStructObj)
% Assign lane parameters from ground-truth lane boundaries.


% Find ego-vehicle lane boundary indices
lbNum = [1, 1];
for j = 1:length(lanesTruth.LaneBoundaries)-1
    yleftLane = lanesTruth.LaneBoundaries(j+1).Coordinates(1,2);
    yrightLane = lanesTruth.LaneBoundaries(j).Coordinates(1,2);
    
    if ((0 >= yleftLane) && (0 <= yrightLane))
        lbNum(1) = j;
        lbNum(2) = j+1;
        break;
    elseif ((0 >= yrightLane) && (0 <= yleftLane))
        lbNum(1) = j+1;
        lbNum(2) = j;
        break;
    end
end

% Assign lane boundaries struct object to output variable
ego_lane_boundaries = boundariesStructObj;

% Assign left lane boundary to output bus, ego_lane_boundaries
ego_lane_boundaries.LaneBoundaries(1) = lanesTruth.LaneBoundaries(lbNum(1));

% Update the left lateral offset value when it is zero to NaN to be
% consistent with Scenario Reader output
if (ego_lane_boundaries.LaneBoundaries(1).LateralOffset == 0)
    ego_lane_boundaries.LaneBoundaries(1).LateralOffset = NaN;
end

% Assign right lane boundary to output bus, ego_lane_boundaries
ego_lane_boundaries.LaneBoundaries(2) = lanesTruth.LaneBoundaries(lbNum(2));

% Update the right lateral offset value when it is zero to NaN to be
% consistent with Scenario Reader output
if (ego_lane_boundaries.LaneBoundaries(2).LateralOffset == 0)
    ego_lane_boundaries.LaneBoundaries(2).LateralOffset = NaN;
end

end

== matlab function HighwayLaneFollowingRRTestBench/Metrics Assessment/MATLAB Function ==
  data: bboxes input; bboxOut output; camera parameter; range parameter
function bboxOut =  filterGroundTruthOutOfRange(bboxes,camera,range)
    % filterGroundTruthOutOfRange Finds the the bounding boxes of actors,
    % that are outside the specified range and filter them from the truth. 
    % This helps in evaluating the vehicle detector at specified ranges,
    % instead of the entire scene. 
    
    % Define Mono Camera sensor
    persistent sensor;
    if isempty(sensor)
        % Compute the camera intrinsics
        camIntrinsics = cameraIntrinsics(camera.FocalLength,camera.PrincipalPoint, camera.ImageSize);
        % Initialize the monocamera sensor
        sensor = monoCamera(camIntrinsics, camera.Position(3),'Pitch', camera.Rotation(2));
    end
    
    % Compute distance in vehicle coordinates.
    bboxOut = zeros(20,4);
    j = 1;
    for i = 1:size(bboxes, 1)
        bbox  = bboxes(i, :);
        if bbox(3)>0 && bbox(4)>0
            yBottom = bbox(2) + bbox(4) - 1;
            xCenter = bbox(1) + (bbox(3)-1)/2;

            %Get the location of the vehicle. 
            location = imageToVehicle(sensor, [xCenter, yBottom]);
    
            % Append the box to the result only if the current vehicle is 
            % within the specified range. 
            if norm(location)<range
                bboxOut(j,:) = bbox;
                j = j+1;
            end
        end
    end

end
